simulink library "qcatlib"  (R2018a)
settings: Solver=VariableStepAuto  StartTime=0.0  StopTime=10.0  RelTol=1e-3
undefined symbols (not defined in the file or in its folder): dyn_ca_sl, qp_ca_sl
settings Model: ExtModeAutoUpdateStatusClock=off  Creator=ola  LastModifiedBy=mengc
settings DataIOCC: SaveFormat=Array  SignalLoggingSaveFormat=ModelDataLogs
settings OptimizationCC: BlockReduction=off  BooleanDataType=off
settings DebuggingCC: SaveWithParameterizedLinksMsg=none  UnderspecifiedInitializationDetection=Classic  MergeDetectMultiDrivingBlocksExec=none  SignalResolutionControl=TryResolveAllWithWarning  MultiTaskDSMMsg=warning  MultiTaskCondExecSysMsg=none
settings HardwareCC: ProdBitPerPointer=32  ProdBitPerSizeT=32  ProdBitPerPtrDiffT=32  ProdLargestAtomicFloat=None  ProdIntDivRoundTo=Undefined  ProdEndianess=Unspecified  ProdWordSize=32  ProdHWDeviceType=32-bit Generic  TargetUnknown=on
settings ModelReferenceCC: PropagateSignalLabelsOutOfModel=off
settings ConfigComp: CovMetricSettings=dw  CovHtmlReporting=on  CovSaveCumulativeToWorkspaceVar=on  CovSaveSingleToWorkspaceVar=on  CovExternalEMLEnable=off

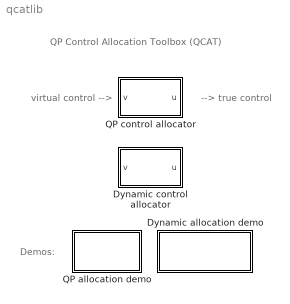
== system qcatlib ==
  note: virtual control -->
  note: --> true control
  note: QP Control Allocation Toolbox (QCAT)
  note: Demos:
  Dynamic allocation demo : Subsystem  mask{A=0}
      mask prompts: A "Needed for OpenSys to work from browser"
      settings: OpenFcn=open_system('dyn_alloc_demo')
      mask Display: disp('Dynamic control\nallocation')
  Dynamic control allocator : Subsystem  mask(Dynamic control allocator){B=[], plim=[], rlim=[], T=1, Wv=[], W1=[], W2=[], S=[]}
      mask prompts: B "Control effectiveness matrix, B"; plim "Position limits, plim"; rlim "Rate limits, rlim"; T "Sampling time, T"; Wv "Virtual control weighting matrix, Wv"; W1 "Control position weighting matrix, W1"; W2 "Control rate weighting matrix, W2"; S "Steady state distribution, S"
      mask help: Given the virtual control command v, the control input u is computed using dynamic control allocation (see help dyn_sim).
      mask Help: See the documentation for dyn_sim.
      mask Display: disp('Dynamic\nCA')
  QP allocation demo : Subsystem  mask{A=0}
      mask prompts: A "Needed for OpenSys to work from browser"
      settings: OpenFcn=open_system('qp_alloc_demo')
      mask Display: disp('QP control\nallocation')
  QP control allocator : Subsystem  AncestorBlock=qcatlib/Dynamic control allocator  mask(QP control allocator){B=[], plim=[], rlim=[], T=1, Wv=[], Wu=[], ud=[], alg=SLS, imax=100, gam=1e4, tol=1e-4}
      mask prompts: B "Control effectiveness matrix, B"; plim "Position limits, plim"; rlim "Rate limits, rlim"; T "Sampling time, T"; Wv "Virtual control weighting matrix, Wv"; Wu "Control weighting matrix, Wu"; ud "Desired control, ud"; alg "Algorithm"; imax "Max no. of iterations"; gam "Weight, gamma"; tol "Tolerance, tol"
      mask help: Given the virtual control command v, the control input u is computed using l2-optimal control allocation (see help qp_sim).
      mask Help: See the documentation for qp_sim.
      mask TypeOptions alg: SLS | WLS | WLSC | MLS | IP | CGI | FXP
      mask Callback alg:
      | val = get_param(gcb,'MaskValues');
      | switch lower(val{8})
      |  case {'sls','mls','cgi'}
      |   set_param(gcb,'MaskVisibilities',{'on','on','on','on','on','on','on','on','on','off','off'});
      |  case {'wls','wlsc','fxp'}
      |   set_param(gcb,'MaskVisibilities',{'on','on','on','on','on','on','on','on','on','on','off'});
      |  case {'ip'}
      |   set_param(gcb,'MaskVisibilities',{'on','on','on','on','off','off','on','on','on','on','on'});
      | end
      mask Display: fprintf('%s',upper(alg))

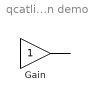
== system qcatlib/Dynamic allocation demo ==
  Gain : Gain  SaturateOnIntegerOverflow=on  OutDataTypeStr=Inherit: Same as input  ParamDataTypeStr=Inherit: Same as input
  wires:
  ? -> Gain/1
  Gain/1 -> ?

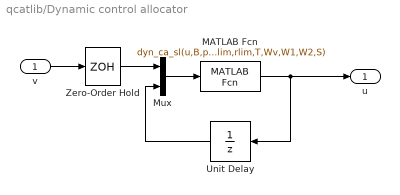
== system qcatlib/Dynamic control allocator ==
  v : Inport
  MATLAB Fcn : MATLABFcn  MATLABFcn=dyn_ca_sl(u,B,plim,rlim,T,Wv,W1,W2,S)  OutputDimensions=size(B,2)
  Mux : Mux  Inputs=2
  Unit Delay : UnitDelay  SampleTime=T
  Zero-Order Hold : ZeroOrderHold  SampleTime=T
  u : Outport
  wires:
  Unit Delay/1 -> Mux/2
  Mux/1 -> MATLAB Fcn/1
  Zero-Order Hold/1 -> Mux/1
  MATLAB Fcn/1 -> Unit Delay/1, u/1
  v/1 -> Zero-Order Hold/1

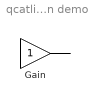
== system qcatlib/QP allocation demo ==
  Gain : Gain  SaturateOnIntegerOverflow=on  OutDataTypeStr=Inherit: Same as input  ParamDataTypeStr=Inherit: Same as input
  wires:
  ? -> Gain/1
  Gain/1 -> ?

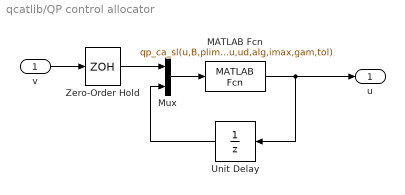
== system qcatlib/QP control allocator ==
  v : Inport
  MATLAB Fcn : MATLABFcn  MATLABFcn=qp_ca_sl(u,B,plim,rlim,T,Wv,Wu,ud,alg,imax,gam,tol)  OutputDimensions=size(B,2)
  Mux : Mux  Inputs=2
  Unit Delay : UnitDelay  SampleTime=T
  Zero-Order Hold : ZeroOrderHold  SampleTime=T
  u : Outport
  wires:
  v/1 -> Zero-Order Hold/1
  Unit Delay/1 -> Mux/2
  Mux/1 -> MATLAB Fcn/1
  Zero-Order Hold/1 -> Mux/1
  MATLAB Fcn/1 -> u/1, Unit Delay/1
